simulink model "SingleWksWithCountBasedSetups"  (R2015a)
settings: Solver=ode45  SolverMode=SingleTasking  StartTime=0.0  StopTime=50000  RelTol=1e-3
InitFcn:
  | se_randomizeseeds(gcs, 'Mode', 'All')
undefined symbols (not defined in the file): se_randomizeseeds
libraries: simeventslib x8
settings Model: CovSFcnEnable=off  Creator=gthiers3  LastModifiedBy=gthiers3
settings OptimizationCC: BlockReduction=off  BooleanDataType=off
settings DebuggingCC: SaveWithParameterizedLinksMsg=none  UnderspecifiedInitializationDetection=Classic  MergeDetectMultiDrivingBlocksExec=none  SignalResolutionControl=TryResolveAllWithWarning
settings HardwareCC: TargetUnknown=on

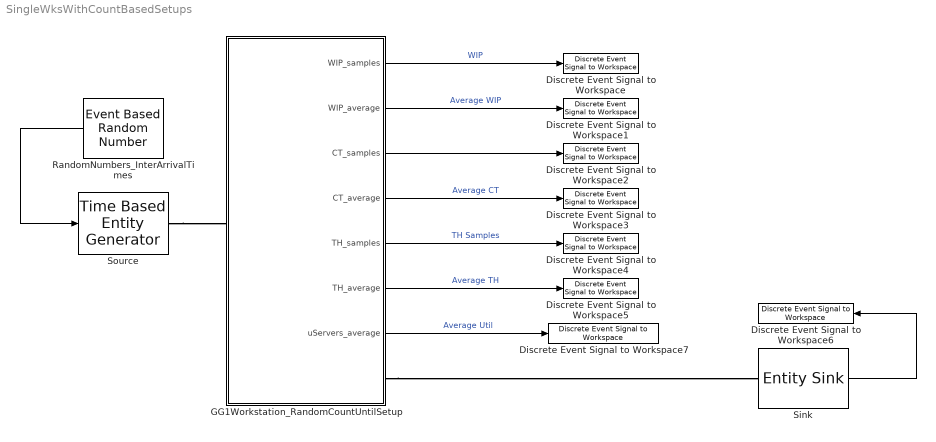
== system SingleWksWithCountBasedSetups ==
  Discrete Event Signal to Workspace : simeventslib/SimEvents Sinks/Discrete Event Signal to Workspace  VariableName=WIP_samples  SaveFormat=Structure With Time  isMonitorOnly=off  isRecordIC=off
  Discrete Event Signal to Workspace1 : simeventslib/SimEvents Sinks/Discrete Event Signal to Workspace  VariableName=WIP_average  SaveFormat=Structure With Time  isMonitorOnly=off  isRecordIC=off
  Discrete Event Signal to Workspace2 : simeventslib/SimEvents Sinks/Discrete Event Signal to Workspace  VariableName=CT_samples  SaveFormat=Structure With Time  isMonitorOnly=off  isRecordIC=off
  Discrete Event Signal to Workspace3 : simeventslib/SimEvents Sinks/Discrete Event Signal to Workspace  VariableName=CT_average  SaveFormat=Structure With Time  isMonitorOnly=off  isRecordIC=off
  Discrete Event Signal to Workspace4 : simeventslib/SimEvents Sinks/Discrete Event Signal to Workspace  VariableName=TH_samples  SaveFormat=Structure With Time  isMonitorOnly=off  isRecordIC=off
  Discrete Event Signal to Workspace5 : simeventslib/SimEvents Sinks/Discrete Event Signal to Workspace  VariableName=TH_average  SaveFormat=Structure With Time  isMonitorOnly=off  isRecordIC=off
  Discrete Event Signal to Workspace6 : simeventslib/SimEvents Sinks/Discrete Event Signal to Workspace  VariableName=nDepartures  SaveFormat=Structure With Time  isMonitorOnly=off  isRecordIC=off
  Discrete Event Signal to Workspace7 : simeventslib/SimEvents Sinks/Discrete Event Signal to Workspace  VariableName=uServers_average  SaveFormat=Structure With Time  isMonitorOnly=off  isRecordIC=off
  GG1Workstation_RandomCountUntilSetup : Subsystem  InitFcn=se_randomizeseeds(gcs, 'Mode', 'All')
      settings: CopyFcn=set_param(gcb, 'LinkStatus', 'none');
  RandomNumbers_InterArrivalTimes : EventBasedRandomNumber  meanExp=1.5  scaleGam=10  meanNorm=100  stdNorm=eps  Seed=17969
  Sink : EntitySink  StatNumberArrived=on
  Source : TimeBasedEntityGenerator  GenerateEntitiesUpon=Intergeneration time from port t
  wires:
  RandomNumbers_InterArrivalTimes/1 -> Source/1
  GG1Workstation_RandomCountUntilSetup/1(WIP_samples) -> Discrete Event Signal to Workspace/1  "WIP"
  GG1Workstation_RandomCountUntilSetup/2(WIP_average) -> Discrete Event Signal to Workspace1/1  "Average WIP"
  GG1Workstation_RandomCountUntilSetup/3(CT_samples) -> Discrete Event Signal to Workspace2/1
  GG1Workstation_RandomCountUntilSetup/4(CT_average) -> Discrete Event Signal to Workspace3/1  "Average CT"
  GG1Workstation_RandomCountUntilSetup/7(uServers_average) -> Discrete Event Signal to Workspace7/1  "Average Util"
  GG1Workstation_RandomCountUntilSetup/6(TH_average) -> Discrete Event Signal to Workspace5/1  "Average TH"
  GG1Workstation_RandomCountUntilSetup/5(TH_samples) -> Discrete Event Signal to Workspace4/1  "TH Samples"
  Sink/1 -> Discrete Event Signal to Workspace6/1
  connections:
  Source/RConn1 -- GG1Workstation_RandomCountUntilSetup/LConn1
  GG1Workstation_RandomCountUntilSetup/RConn1 -- Sink/LConn1

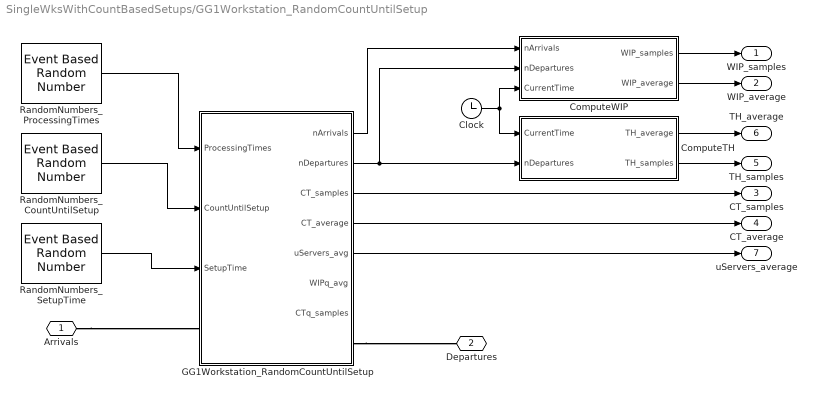
== system SingleWksWithCountBasedSetups/GG1Workstation_RandomCountUntilSetup ==
  Clock : Clock
  ComputeTH : Subsystem
  ComputeWIP : Subsystem
  GG1Workstation_RandomCountUntilSetup : Subsystem
      mask DialogControl DescTextVar Prompt: GG1 Workstation, with a random count of entities serviced until a setup, and random setup times.  Setups are functionally equivalent to any non-preemptive (e.g. non-interrupting) downtime, for example preventative maintenance.
  RandomNumbers_CountUntilSetup : EventBasedRandomNumber  Distribution=Geometric  meanExp=10  minUnif=40  maxUnif=40  pOneBern=40  pSuccessBino=40  numTrialBino=40  minTri=10  maxTri=10  modeTri=10  scaleGam=166.6667  shapeGam=0.72  meanNorm=1000  stdNorm=1.4901e-08  pSuccessGeo=1/11  meanPoiss=10  thresholdLogn=40  scaleLogn=40  shapeLogn=40  thresholdLogl=40  scaleLogl=40  minBeta=40  maxBeta=40  shape1Beta=40  shape2Beta=40  minUnid=40  maxUnid=40  numValueUnid=40  thresholdWbl=40  scaleWbl=40  shapeWbl=40  valueVecCont=40  cdfVecCont=40  valueVecDisc=40  probVecDisc=40  Seed=60986
  RandomNumbers_ProcessingTimes : EventBasedRandomNumber  Distribution=Triangular  minUnif=40  maxUnif=40  pOneBern=40  pSuccessBino=40  numTrialBino=40  minTri=0.4  maxTri=1.4  modeTri=1.35  thresholdGam=40  scaleGam=40  shapeGam=40  meanNorm=95  stdNorm=eps  pSuccessGeo=40  meanPoiss=40  thresholdLogn=40  scaleLogn=40  shapeLogn=40  thresholdLogl=40  scaleLogl=40  minBeta=40  maxBeta=40  shape1Beta=40  shape2Beta=40  minUnid=40  maxUnid=40  numValueUnid=40  thresholdWbl=40  scaleWbl=40  shapeWbl=40  valueVecCont=40  cdfVecCont=40  valueVecDisc=40  probVecDisc=40  Seed=11535
  RandomNumbers_SetupTime : EventBasedRandomNumber  meanExp=2  minUnif=40  maxUnif=40  pOneBern=40  pSuccessBino=40  numTrialBino=40  minTri=38  maxTri=38  modeTri=38  scaleGam=20  meanNorm=eps  stdNorm=eps  meanPoiss=40  thresholdLogn=40  scaleLogn=40  shapeLogn=40  thresholdLogl=40  scaleLogl=40  minBeta=40  maxBeta=40  shape1Beta=40  shape2Beta=40  minUnid=40  maxUnid=40  numValueUnid=40  thresholdWbl=40  scaleWbl=40  shapeWbl=40  valueVecCont=40  cdfVecCont=40  probVecDisc=[0 1]  Seed=14752
  Arrivals : PMIOPort  Port=1  Side=Left
  Departures : PMIOPort  Port=2  Side=Right
  WIP_samples : Outport
  WIP_average : Outport  Port=2
  CT_samples : Outport  Port=3
  CT_average : Outport  Port=4
  TH_samples : Outport  Port=5
  TH_average : Outport  Port=6
  uServers_average : Outport  Port=7
  wires:
  GG1Workstation_RandomCountUntilSetup/2(nDepartures) -> ComputeTH/2(nDepartures), ComputeWIP/2(nDepartures)
  GG1Workstation_RandomCountUntilSetup/3(CT_samples) -> CT_samples/1
  ComputeWIP/1(WIP_samples) -> WIP_samples/1
  GG1Workstation_RandomCountUntilSetup/1(nArrivals) -> ComputeWIP/1(nArrivals)
  Clock/1 -> ComputeWIP/3(CurrentTime), ComputeTH/1(CurrentTime)
  ComputeTH/1(TH_average) -> TH_average/1
  ComputeTH/2(TH_samples) -> TH_samples/1
  RandomNumbers_CountUntilSetup/1 -> GG1Workstation_RandomCountUntilSetup/2(CountUntilSetup)
  RandomNumbers_SetupTime/1 -> GG1Workstation_RandomCountUntilSetup/3(SetupTime)
  RandomNumbers_ProcessingTimes/1 -> GG1Workstation_RandomCountUntilSetup/1(ProcessingTimes)
  GG1Workstation_RandomCountUntilSetup/5(uServers_avg) -> uServers_average/1
  GG1Workstation_RandomCountUntilSetup/4(CT_average) -> CT_average/1
  ComputeWIP/2(WIP_average) -> WIP_average/1
  connections:
  GG1Workstation_RandomCountUntilSetup/RConn1 -- Departures/RConn1
  Arrivals/RConn1 -- GG1Workstation_RandomCountUntilSetup/LConn1

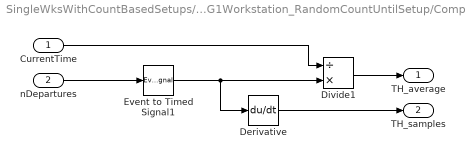
== system SingleWksWithCountBasedSetups/GG1Workstation_RandomCountUntilSetup/ComputeTH ==
  CurrentTime : Inport
  nDepartures : Inport  Port=2
  Derivative : Derivative
  Divide1 : Product  Inputs=/*
  Event to Timed Signal1 : EventToTimedSignal
  TH_average : Outport
  TH_samples : Outport  Port=2
  wires:
  CurrentTime/1 -> Divide1/1
  Event to Timed Signal1/1 -> Derivative/1, Divide1/2
  Divide1/1 -> TH_average/1
  Derivative/1 -> TH_samples/1
  nDepartures/1 -> Event to Timed Signal1/1

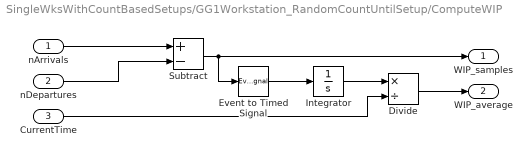
== system SingleWksWithCountBasedSetups/GG1Workstation_RandomCountUntilSetup/ComputeWIP ==
  nArrivals : Inport
  nDepartures : Inport  Port=2
  CurrentTime : Inport  Port=3
  Divide : Product  Inputs=*/
  Event to Timed Signal : EventToTimedSignal
  Integrator : Integrator
  Subtract : Sum  Inputs=+-
  WIP_samples : Outport
  WIP_average : Outport  Port=2
  wires:
  Subtract/1 -> WIP_samples/1, Event to Timed Signal/1
  Event to Timed Signal/1 -> Integrator/1
  Divide/1 -> WIP_average/1
  Integrator/1 -> Divide/1
  nArrivals/1 -> Subtract/1
  nDepartures/1 -> Subtract/2
  CurrentTime/1 -> Divide/2

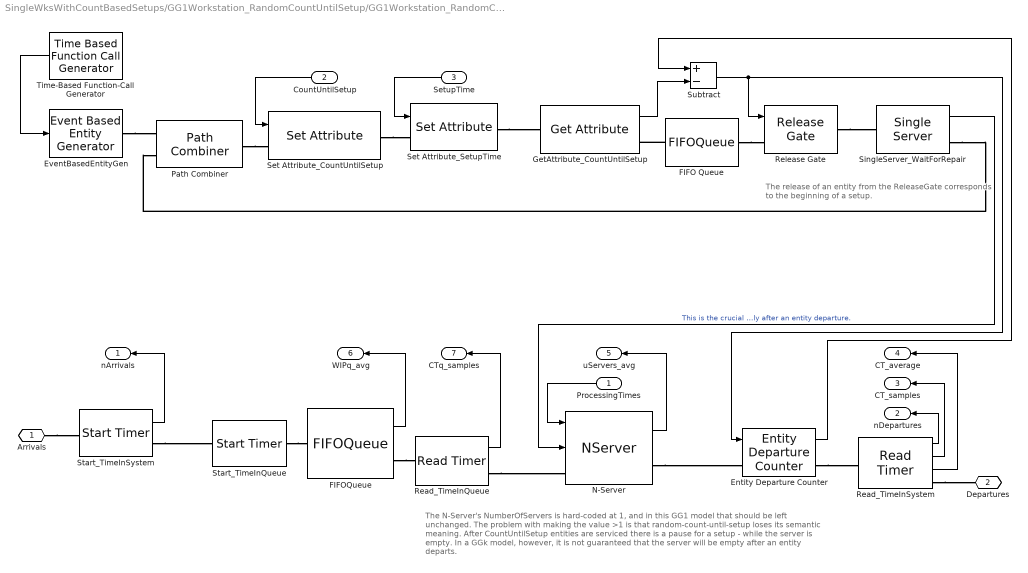
== system SingleWksWithCountBasedSetups/GG1Workstation_RandomCountUntilSetup/GG1Workstation_RandomCountUntilSetup ==
  note: The release of an entity from the ReleaseGate
      | corresponds to the beginning of a setup.
  note: The N-Server's NumberOfServers is hard-coded at 1, and in this GG1 model
      | that should be left unchanged.  The problem with making the value >1 is that
      | random-count-until-setup loses its semantic meaning.  After CountUntilSetup
      | entities are serviced there is a pause for a setup - while the server is empty.  In
      | a GGk model, however, it is not guaranteed that the server will be empty after
      | an entity departs.
  ProcessingTimes : Inport
  CountUntilSetup : Inport  Port=2
  SetupTime : Inport  Port=3
  Entity Departure Counter : EntityDepartureCounter  NumberDepartedToSignal=on  NumberDepartedToAttribute=off  CounterResetTypeOption=Trigger from port tr
  EventBasedEntityGen : EventBasedEntityGenerator  GenerateEntitiesUpon=Function call from port fcn
  FIFO Queue : FIFOQueue  Capacity=Inf
  FIFOQueue : FIFOQueue  Capacity=Inf  StatAverageQueueLength=on
      settings: OutputPortMap=o3
  GetAttribute_CountUntilSetup : GetAttribute  AttributeName=CountUntilSetup  EvaluatedDefaultAttributeValue={ []}
      settings: OutputPortMap=o1
  N-Server : NServer  NumberOfServers=1  ServiceTimeFrom=Signal port t  AllowServiceControl=on  BlockWhileSignalOn=on  StatUtilization=on
      settings: InputPortMap=u0,u1  OutputPortMap=o5
  Path Combiner : PathCombiner  NumberInputPorts=2
  Read_TimeInQueue : ReadTimer  TimerTag=TimeInQueue  StatTimeElapsed=on
      settings: OutputPortMap=o2
  Read_TimeInSystem : ReadTimer  TimerTag=TimeInSystem  StatNumberDeparted=on  StatTimeElapsed=on  StatAverageTimeElapsed=on
      settings: OutputPortMap=o0,o2,o3
  Release Gate : ReleaseGate  OpenGateUpon=Trigger from port tr
  Set Attribute_CountUntilSetup : SetAttribute  AttributeName=CountUntilSetup  AttributeFrom=Signal port  EvaluatedAttributeValue={ []}
  Set Attribute_SetupTime : SetAttribute  AttributeName=SetupTime  AttributeFrom=Signal port  EvaluatedAttributeValue={ []}
  SingleServer_WaitForRepair : SingleServer  ServiceTimeFrom=Attribute  AttributeName=SetupTime  StatNumberInBlock=on
      settings: OutputPortMap=o1
  Start_TimeInQueue : StartTimer  TimerTag=TimeInQueue  TimerStartedOption=Restart
  Start_TimeInSystem : StartTimer  TimerTag=TimeInSystem  TimerStartedOption=Restart  StatNumberDeparted=on
  Subtract : Sum  Inputs=+-
  Time-Based Function-Call Generator : TimeBasedFunctionCallGenerator  EventGenerationMode=Only at simulation start
  Arrivals : PMIOPort  Port=1  Side=Left
  Departures : PMIOPort  Port=2  Side=Right
  nArrivals : Outport
  nDepartures : Outport  Port=2
  CT_samples : Outport  Port=3
  CT_average : Outport  Port=4
  uServers_avg : Outport  Port=5
  WIPq_avg : Outport  Port=6
  CTq_samples : Outport  Port=7
  wires:
  Read_TimeInSystem/2 -> CT_samples/1
  N-Server/1 -> uServers_avg/1
  Read_TimeInQueue/1 -> CTq_samples/1
  FIFOQueue/1 -> WIPq_avg/1
  Start_TimeInSystem/1 -> nArrivals/1
  Read_TimeInSystem/1 -> nDepartures/1
  ProcessingTimes/1 -> N-Server/1
  Read_TimeInSystem/3 -> CT_average/1
  SetupTime/1 -> Set Attribute_SetupTime/1
  Time-Based Function-Call Generator/1 -> EventBasedEntityGen/1
  CountUntilSetup/1 -> Set Attribute_CountUntilSetup/1
  Subtract/1 -> Entity Departure Counter/1, Release Gate/1
  GetAttribute_CountUntilSetup/1 -> Subtract/2
  Entity Departure Counter/1 -> Subtract/1
  SingleServer_WaitForRepair/1 -> N-Server/2  "This is the crucial blocking signal; when > 0 the N-Server will be preemptively disabled. Non-preemption in this model is an approximation, because disabling of the N-Server  should follow shortly after an entity departure."
  connections:
  Arrivals/RConn1 -- Start_TimeInSystem/LConn1
  FIFOQueue/RConn1 -- Read_TimeInQueue/LConn1
  Start_TimeInSystem/RConn1 -- Start_TimeInQueue/LConn1
  Read_TimeInSystem/RConn1 -- Departures/RConn1
  Read_TimeInQueue/RConn1 -- N-Server/LConn1
  Start_TimeInQueue/RConn1 -- FIFOQueue/LConn1
  Path Combiner/RConn1 -- Set Attribute_CountUntilSetup/LConn1
  EventBasedEntityGen/RConn1 -- Path Combiner/LConn1
  SingleServer_WaitForRepair/RConn1 -- Path Combiner/LConn2
  Set Attribute_CountUntilSetup/RConn1 -- Set Attribute_SetupTime/LConn1
  N-Server/RConn1 -- Entity Departure Counter/LConn1
  Entity Departure Counter/RConn1 -- Read_TimeInSystem/LConn1
  Set Attribute_SetupTime/RConn1 -- GetAttribute_CountUntilSetup/LConn1
  FIFO Queue/LConn1 -- GetAttribute_CountUntilSetup/RConn1
  Release Gate/RConn1 -- SingleServer_WaitForRepair/LConn1
  FIFO Queue/RConn1 -- Release Gate/LConn1
